simulink model "trig_03"  (R2022a)
settings: Solver=VariableStepDiscrete  StartTime=0.0  StopTime=20.0  RelTol=1e-3
libraries: simulink x2
settings Model: Creator=FUGAZI  LastModifiedBy=FUGAZI

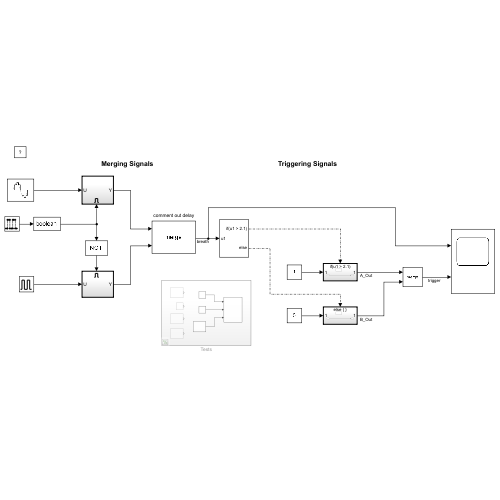
[thumbnail: Simulink's stored preview of the top-level diagram]
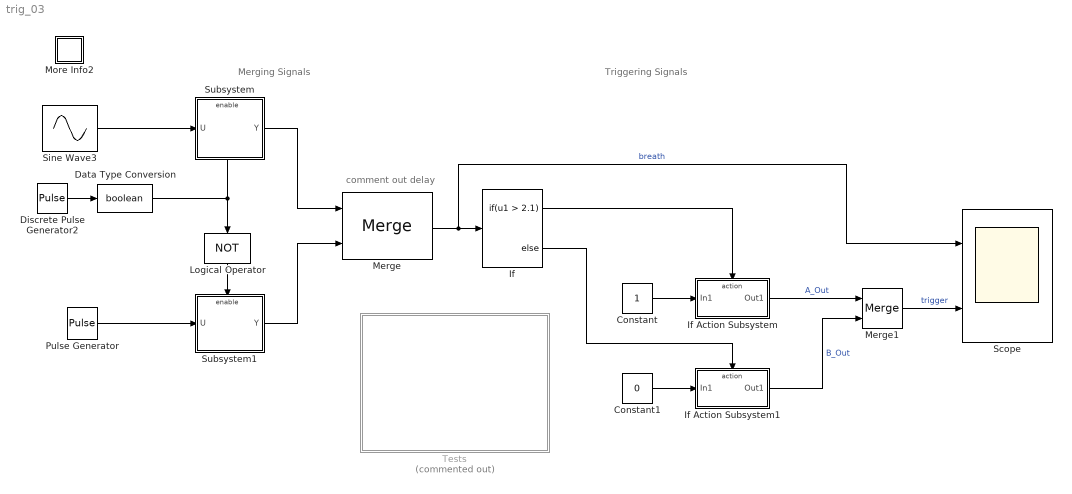
== system trig_03 ==
  note: comment out delay
  note: Merging Signals
  note: Triggering Signals
  Constant : Constant
  Constant1 : Constant  Value=0
  Data Type Conversion : DataTypeConversion  OutDataTypeStr=boolean
  Discrete Pulse Generator2 : DiscretePulseGenerator  Period=8  PhaseDelay=7  SampleTime=0.25
  If : If  IfExpression=u1 > 2.1
  If Action Subsystem : Subsystem  TreatAsAtomicUnit=on
  If Action Subsystem1 : Subsystem  TreatAsAtomicUnit=on
  Logical Operator : Logic  Operator=NOT  Inputs=1  OutDataTypeStr=boolean
  Merge : Merge
  Merge1 : Merge
  More Info2 : Subsystem
      settings: OpenFcn=showExample('simulink_features/MergingSignalsExample')
      mask Display: disp('?')
  Pulse Generator : DiscretePulseGenerator  PulseType=Time based  Amplitude=2  PulseWidth=40  PhaseDelay=3
  Scope : Scope  NumInputPorts=2
  Sine Wave3 : Sin  Amplitude=2.2  Frequency=3.14  Phase=2.365  Samples=2  SampleTime=0.05
  Subsystem : Subsystem  Tag=MergeExample  TreatAsAtomicUnit=on
  Subsystem1 : Subsystem  Tag=MergeExample  TreatAsAtomicUnit=on
  Tests : Subsystem  Commented=on
  wires:
  Merge/1 -> Scope/1, If/1  "breath"
  Subsystem/1(Y) -> Merge/1
  Logical Operator/1 -> Subsystem1/Enable
  Data Type Conversion/1 -> Logical Operator/1, Subsystem/Enable
  Discrete Pulse Generator2/1 -> Data Type Conversion/1
  Subsystem1/1(Y) -> Merge/2
  Pulse Generator/1 -> Subsystem1/1(U)
  Sine Wave3/1 -> Subsystem/1(U)
  If Action Subsystem/1(Out1) -> Merge1/1  "A_Out"
  If/2 -> If Action Subsystem1/Action
  If Action Subsystem1/1(Out1) -> Merge1/2  "B_Out"
  Constant/1 -> If Action Subsystem/1(In1)
  Constant1/1 -> If Action Subsystem1/1(In1)
  If/1 -> If Action Subsystem/Action
  Merge1/1 -> Scope/2  "trigger"

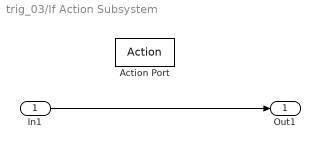
== system trig_03/If Action Subsystem ==
  In1 : Inport
  Action Port : ActionPort  ActionPortLabel=if(u1 > 2.1)
  Out1 : Outport
  wires:
  In1/1 -> Out1/1

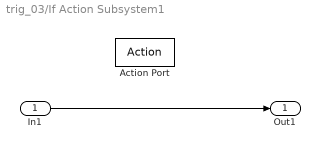
== system trig_03/If Action Subsystem1 ==
  In1 : Inport
  Action Port : ActionPort  ActionPortLabel=else
  Out1 : Outport
  wires:
  In1/1 -> Out1/1

== system trig_03/More Info2 ==

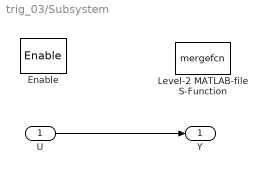
== system trig_03/Subsystem ==
  U : Inport
  Enable : EnablePort  StatesWhenEnabling=reset
  Level-2 MATLAB-file S-Function : M-S-Function  FunctionName=mergefcn
  Y : Outport  VectorParamsAs1DForOutWhenUnconnected=off
  wires:
  U/1 -> Y/1

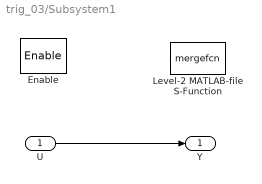
== system trig_03/Subsystem1 ==
  U : Inport
  Enable : EnablePort  StatesWhenEnabling=reset
  Level-2 MATLAB-file S-Function : M-S-Function  FunctionName=mergefcn
  Y : Outport  VectorParamsAs1DForOutWhenUnconnected=off
  wires:
  U/1 -> Y/1

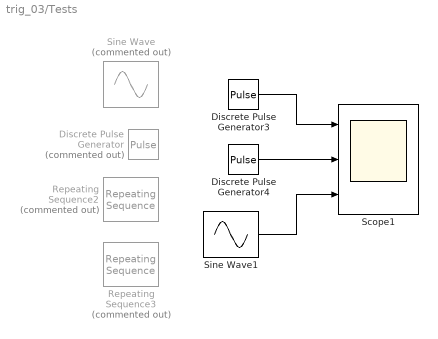
== system trig_03/Tests ==
  Discrete Pulse Generator : DiscretePulseGenerator  Commented=on  SampleTime=5
  Discrete Pulse Generator3 : DiscretePulseGenerator  Period=4  PhaseDelay=3  SampleTime=0.5
  Discrete Pulse Generator4 : DiscretePulseGenerator  SampleTime=2
  Repeating Sequence2 : simulink/Sources/Repeating Sequence  Commented=on  rep_seq_t=[0 0.1 2 2.1 4]  rep_seq_y=[0 2 2 0 0]
  Repeating Sequence3 : simulink/Sources/Repeating Sequence  Commented=on  rep_seq_t=[0 4 4.05 8 8.05]  rep_seq_y=[2 2 0 0 2]
  Scope1 : Scope  NumInputPorts=3
  Sine Wave : Sin  Commented=on  Amplitude=2.2  Frequency=pi  SampleTime=0
  Sine Wave1 : Sin  Amplitude=2.2  Frequency=3.14  Phase=2.365  Samples=2  SampleTime=0.05
  wires:
  Discrete Pulse Generator3/1 -> Scope1/1
  Sine Wave1/1 -> Scope1/3
  Discrete Pulse Generator4/1 -> Scope1/2
